simulink model "p4"  (R2018a)
settings: Solver=VariableStepAuto  StartTime=0.0  StopTime=10.0  RelTol=1e-3
settings Model: Creator=ASUS  LastModifiedBy=ASUS

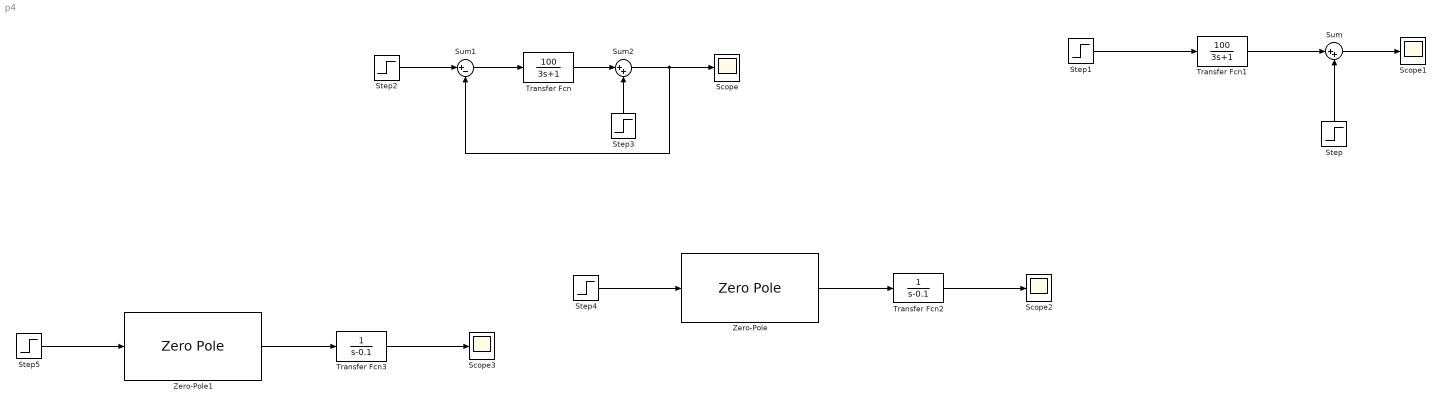
== system p4 ==
  Scope{,1..3} (4 alike) : Scope
  Step : Step  Time=5  After=10  SampleTime=0
  Step1 : Step  Time=0  SampleTime=0
  Step2 : Step  Time=0  SampleTime=0
  Step3 : Step  Time=5  After=10  SampleTime=0
  Step4 : Step  SampleTime=0
  Step5 : Step  SampleTime=0
  Sum : Sum  Inputs=|++
  Sum1 : Sum  Inputs=|+-
  Sum2 : Sum  Inputs=|++
  Transfer Fcn : TransferFcn  Numerator=[100]  Denominator=[3 1]
  Transfer Fcn1 : TransferFcn  Numerator=[100]  Denominator=[3 1]
  Transfer Fcn2 : TransferFcn  Denominator=[1 -0.1]
  Transfer Fcn3 : TransferFcn  Denominator=[1 -0.1]
  Zero-Pole : ZeroPole  Zeros=[-0.099]  Poles=-8
  Zero-Pole1 : ZeroPole  Zeros=[0.1]  Poles=-8
  wires:
  Step1/1 -> Transfer Fcn1/1
  Transfer Fcn1/1 -> Sum/1
  Sum/1 -> Scope1/1
  Step/1 -> Sum/2
  Sum1/1 -> Transfer Fcn/1
  Step2/1 -> Sum1/1
  Transfer Fcn/1 -> Sum2/1
  Step3/1 -> Sum2/2
  Sum2/1 -> Sum1/2, Scope/1
  Zero-Pole/1 -> Transfer Fcn2/1
  Step4/1 -> Zero-Pole/1
  Transfer Fcn2/1 -> Scope2/1
  Step5/1 -> Zero-Pole1/1
  Transfer Fcn3/1 -> Scope3/1
  Zero-Pole1/1 -> Transfer Fcn3/1
